simulink model "QuarterCar_ActiveSusp_KF_Simulink2018b"  (R2018b)
settings: Solver=ode4  StartTime=0.0  StopTime=SIM_TIME  FixedStep=STEP_SIZE  RelTol=1e-3
undefined symbols (not defined in the file or in its folder): b_s, b_t, C_kf, F_kf, G_kf, k_s, k_t, L_kf, m_s, m_u, Ts, V2d, x0hat
settings Model: Creator=Roberto  LastModifiedBy=Roberto

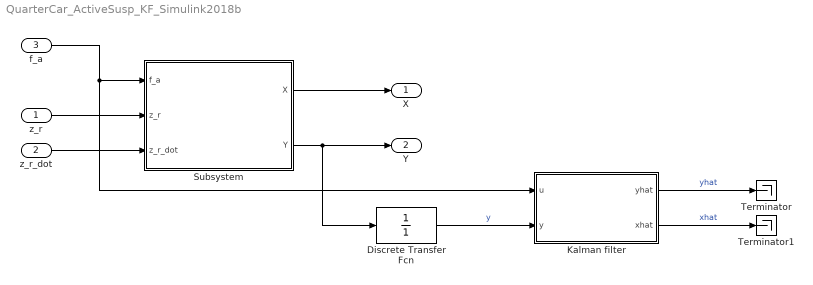
== system QuarterCar_ActiveSusp_KF_Simulink2018b ==
  z_r : Inport
  z_r_dot : Inport  Port=2
  f_a : Inport  Port=3
  Discrete Transfer Fcn : DiscreteTransferFcn  Denominator=[1]  SampleTime=Ts
  Kalman filter : Subsystem
  Subsystem : Subsystem
  Terminator : Terminator
  Terminator1 : Terminator
  X : Outport
  Y : Outport  Port=2
  wires:
  f_a/1 -> Kalman filter/1(u), Subsystem/1(f_a)
  z_r/1 -> Subsystem/2(z_r)
  z_r_dot/1 -> Subsystem/3(z_r_dot)
  Subsystem/1(X) -> X/1
  Subsystem/2(Y) -> Discrete Transfer Fcn/1, Y/1
  Kalman filter/2(xhat) -> Terminator1/1  "xhat"
  Kalman filter/1(yhat) -> Terminator/1  "yhat"
  Discrete Transfer Fcn/1 -> Kalman filter/2(y)  "y"

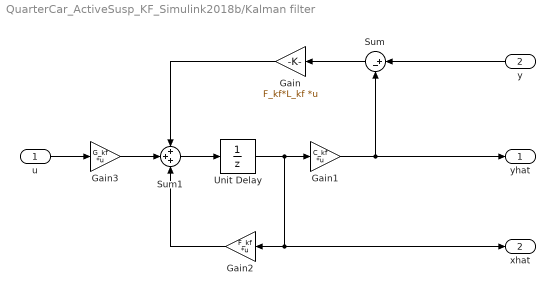
== system QuarterCar_ActiveSusp_KF_Simulink2018b/Kalman filter ==
  u : Inport
  y : Inport  Port=2
  Gain : Gain  Gain=F_kf*L_kf  Multiplication=Matrix(K*u) (u vector)
  Gain1 : Gain  Gain=C_kf  Multiplication=Matrix(K*u) (u vector)
  Gain2 : Gain  Gain=F_kf  Multiplication=Matrix(K*u) (u vector)
  Gain3 : Gain  Gain=G_kf  Multiplication=Matrix(K*u) (u vector)
  Sum : Sum  Inputs=|+-
  Sum1 : Sum  Inputs=+++
  Unit Delay : UnitDelay  InitialCondition=x0hat  SampleTime=Ts
  yhat : Outport
  xhat : Outport  Port=2
  wires:
  Gain3/1 -> Sum1/2
  y/1 -> Sum/1
  Gain/1 -> Sum1/1
  Sum/1 -> Gain/1
  u/1 -> Gain3/1
  Gain2/1 -> Sum1/3
  Sum1/1 -> Unit Delay/1
  Gain1/1 -> yhat/1, Sum/2
  Unit Delay/1 -> xhat/1, Gain2/1, Gain1/1

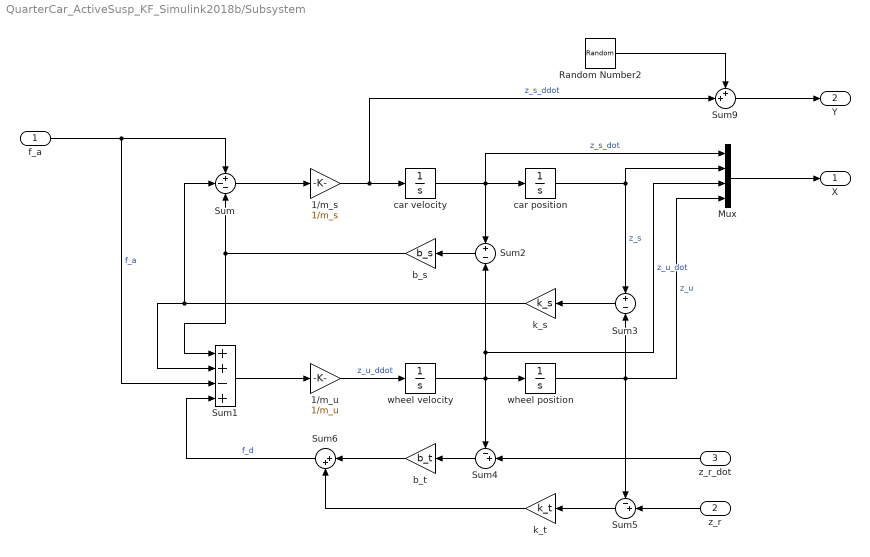
== system QuarterCar_ActiveSusp_KF_Simulink2018b/Subsystem ==
  f_a : Inport
  z_r : Inport  Port=2
  z_r_dot : Inport  Port=3
  1/m_s : Gain  Gain=1/m_s
  1/m_u : Gain  Gain=1/m_u
  Mux : Mux
  Random Number2 : RandomNumber  Variance=V2d  Seed=[5821490]  SampleTime=Ts
  Sum : Sum  Inputs=+--
  Sum1 : Sum  Inputs=++-+
  Sum2 : Sum  Inputs=+-
  Sum3 : Sum  Inputs=+-
  Sum4 : Sum  Inputs=-+|
  Sum5 : Sum  Inputs=-+|
  Sum6 : Sum  Inputs=|++
  Sum9 : Sum  Inputs=++|
  b_s : Gain  Gain=b_s
  b_t : Gain  Gain=b_t
  car position : Integrator
  car velocity : Integrator
  k_s : Gain  Gain=k_s
  k_t : Gain  Gain=k_t
  wheel position : Integrator
  wheel velocity : Integrator
  X : Outport
  Y : Outport  Port=2
  wires:
  wheel velocity/1 -> Sum4/1, Mux/3, Sum2/2, wheel position/1  "z_u_dot"
  Sum1/1 -> 1/m_u/1
  car position/1 -> Mux/2, Sum3/1  "z_s"
  k_s/1 -> Sum/2, Sum1/2
  z_r/1 -> Sum5/2
  1/m_u/1 -> wheel velocity/1  "z_u_ddot"
  Sum6/1 -> Sum1/4  "f_d"
  z_r_dot/1 -> Sum4/2
  Sum3/1 -> k_s/1
  1/m_s/1 -> Sum9/2, car velocity/1  "z_s_ddot"
  Sum2/1 -> b_s/1
  car velocity/1 -> Mux/1, Sum2/1, car position/1  "z_s_dot"
  b_s/1 -> Sum1/1, Sum/3
  b_t/1 -> Sum6/1
  Sum/1 -> 1/m_s/1
  wheel position/1 -> Mux/4, Sum5/1, Sum3/2  "z_u"
  Sum4/1 -> b_t/1
  f_a/1 -> Sum1/3, Sum/1  "f_a"
  k_t/1 -> Sum6/2
  Sum5/1 -> k_t/1
  Mux/1 -> X/1
  Random Number2/1 -> Sum9/1
  Sum9/1 -> Y/1
